simulink model "exaktlin"  (Simulink 10.3)
settings: Solver=ode45  StartTime=0.0  StopTime=100  RelTol=1e-3  EnableMultiTasking=on
values from neighbouring files (symbols this model uses):
  L = place(A, B, p)    [Task5.m]    (also in sbefu.m = length(fun))
  Lr = inv(C*inv(B*L -A)*B)    [Task5.m]
settings Model: Creator=axelsson  LastModifiedBy=emiwi425
settings DataIOCC: LimitDataPoints=on
settings DebuggingCC: SolverPrmCheckMsg=warning

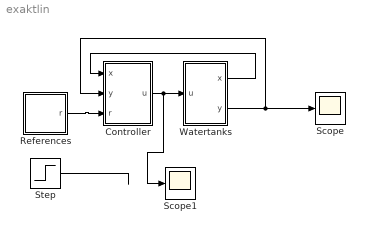
== system exaktlin ==
  Controller : Subsystem
  References : Subsystem  mask{t1=0, r0=5, r1=1}
      mask prompts: t1 "Tid för steget"; r0 "Startnivå"; r1 "Höjd på steget"
  Scope : Scope
  Scope1 : Scope
  Step : Step  SampleTime=0
  Watertanks : Subsystem
  wires:
  Controller/1(u) -> Scope1/1, Watertanks/1(u)
  References/1(r) -> Controller/3(r)
  Watertanks/1(x) -> Controller/1(x)
  Watertanks/2(y) -> Controller/2(y), Scope/1
  Step/1 -> ?

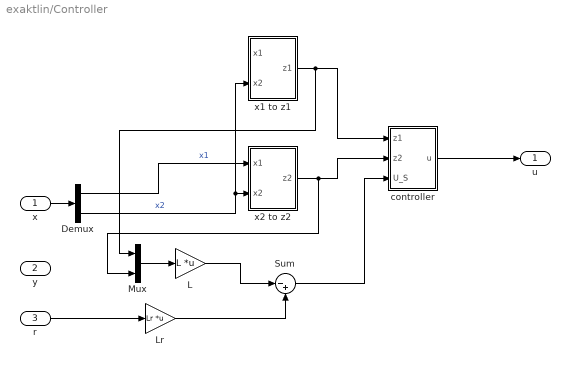
== system exaktlin/Controller ==
  x : Inport
  y : Inport  Port=2
  r : Inport  Port=3
  Demux : Demux  Outputs=2
  L : Gain  Gain=L  Multiplication=Matrix(K*u)
  Lr : Gain  Gain=Lr  Multiplication=Matrix(K*u)
  Mux : Mux  Inputs=2
  Sum : Sum  Inputs=|-+
  controller : Subsystem
  x1 to z1 : Subsystem
  x2 to z2 : Subsystem
  u : Outport
  wires:
  x/1 -> Demux/1
  Demux/2 -> x1 to z1/2(x2), x2 to z2/2(x2)  "x2"
  Demux/1 -> x2 to z2/1(x1)  "x1"
  x2 to z2/1(z2) -> Mux/2, controller/2(z2)
  x1 to z1/1(z1) -> Mux/1, controller/1(z1)
  controller/1(u) -> u/1
  r/1 -> Lr/1
  Mux/1 -> L/1
  L/1 -> Sum/1
  Lr/1 -> Sum/2
  Sum/1 -> controller/3(U_S)

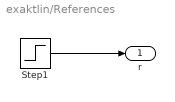
== system exaktlin/References ==
  Step1 : Step  Time=t1  Before=r0  After=r0+r1  SampleTime=0
  r : Outport
  wires:
  Step1/1 -> r/1

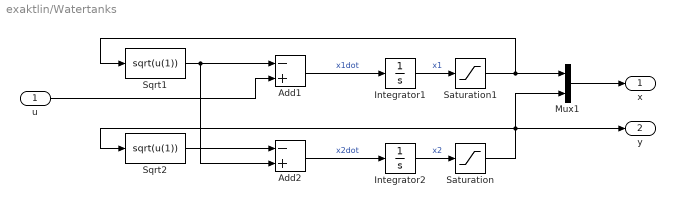
== system exaktlin/Watertanks ==
  u : Inport
  Add1 : Sum  Inputs=-+
  Add2 : Sum  Inputs=-+
  Integrator1 : Integrator  InitialCondition=5
  Integrator2 : Integrator  InitialCondition=5
  Mux1 : Mux  Inputs=2
  Saturation : Saturate  UpperLimit=100  LowerLimit=0
  Saturation1 : Saturate  UpperLimit=100  LowerLimit=0
  Sqrt1 : Fcn  Expr=sqrt(u(1))
  Sqrt2 : Fcn  Expr=sqrt(u(1))
  x : Outport
  y : Outport  Port=2
  wires:
  Integrator1/1 -> Saturation1/1  "x1"
  Integrator2/1 -> Saturation/1  "x2"
  Sqrt2/1 -> Add2/1
  Add2/1 -> Integrator2/1  "x2dot"
  Sqrt1/1 -> Add2/2, Add1/1
  Add1/1 -> Integrator1/1  "x1dot"
  u/1 -> Add1/2
  Mux1/1 -> x/1
  Saturation/1 -> Sqrt2/1, y/1, Mux1/2
  Saturation1/1 -> Sqrt1/1, Mux1/1

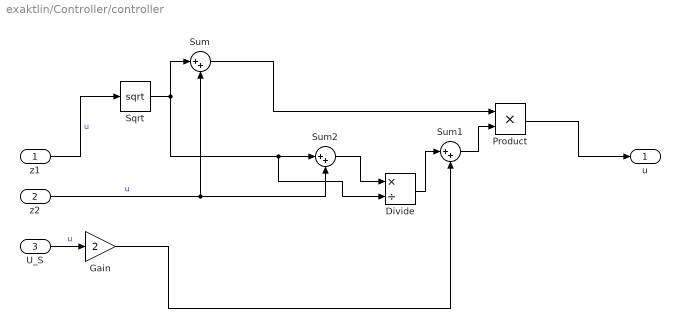
== system exaktlin/Controller/controller ==
  z1 : Inport
  z2 : Inport  Port=2
  U_S : Inport  Port=3
  Divide : Product  Inputs=*/
  Gain : Gain  Gain=2
  Product : Product
  Sqrt : Sqrt  SaturateOnIntegerOverflow=on
  Sum : Sum  Inputs=|++
  Sum1 : Sum  Inputs=|++
  Sum2 : Sum  Inputs=|++
  u : Outport
  wires:
  z1/1 -> Sqrt/1  "u"
  Sqrt/1 -> Divide/2, Sum2/1, Sum/1
  z2/1 -> Sum2/2, Sum/2  "u"
  Sum/1 -> Product/1
  U_S/1 -> Gain/1  "u"
  Gain/1 -> Sum1/2
  Sum2/1 -> Divide/1
  Divide/1 -> Sum1/1
  Sum1/1 -> Product/2
  Product/1 -> u/1

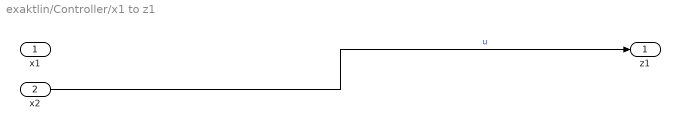
== system exaktlin/Controller/x1 to z1 ==
  x1 : Inport
  x2 : Inport  Port=2
  z1 : Outport
  wires:
  x2/1 -> z1/1  "u"

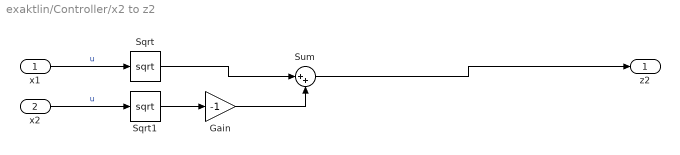
== system exaktlin/Controller/x2 to z2 ==
  x1 : Inport
  x2 : Inport  Port=2
  Gain : Gain  Gain=-1
  Sqrt : Sqrt  SaturateOnIntegerOverflow=on
  Sqrt1 : Sqrt  SaturateOnIntegerOverflow=on
  Sum : Sum  Inputs=|++
  z2 : Outport
  wires:
  x1/1 -> Sqrt/1  "u"
  x2/1 -> Sqrt1/1  "u"
  Sqrt1/1 -> Gain/1
  Gain/1 -> Sum/2
  Sqrt/1 -> Sum/1
  Sum/1 -> z2/1
